simulink model "Lab_RS232_noHFC"  (Simulink 7.8)
settings: Solver=VariableStepDiscrete  StartTime=0.0  StopTime=Inf  FixedStep=Ts/4  RelTol=1e-3
PreLoadFcn:
  | clear all;
  | close all;
  | clc;
  | 
  | Txs = 1;          % Gen clk (period)
  | Trs = 1;           % Sink clk (period)
  | 
  | N = 8;    % No of characters to exchange
StartFcn:
  | clc;
  | close all;
  | 
  | TxBuffer = randi([0 255],1,N);   % Tx characters tmp array
  | RxBuffer = ones(1,N);   % Rx characters tmp array
  | 
  | RS232_Start;
StopFcn:
  | RS232_End;
  | 
  | if size(TxBuffer) == size(RxBuffer)
  |   if TxBuffer == RxBuffer
  |     disp('OK');
  |   else
  |      disp('Error');
  |      plot(TxBuffer-RxBuffer, 'o');
  |   end
  | else
  |      disp('Error: Incorrect No of characters');
  | end
libraries: simulink x1
settings Model: Creator=theodore  LastModifiedBy=theodore
settings DebuggingCC: SolverPrmCheckMsg=none

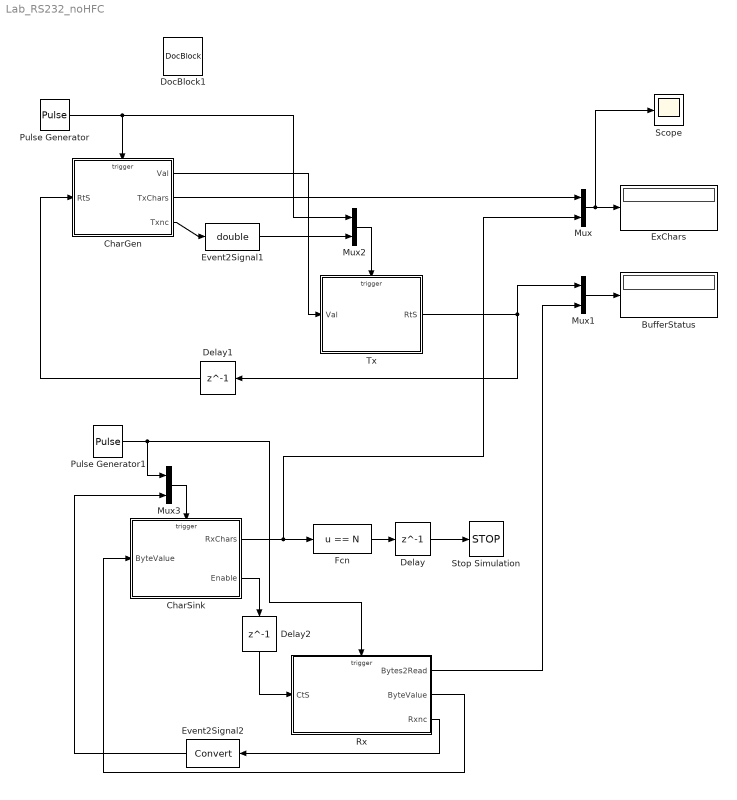
== system Lab_RS232_noHFC ==
  BufferStatus : Display
  CharGen : Stateflow chart  TreatAsAtomicUnit=on
  CharSink : Stateflow chart  TreatAsAtomicUnit=on
  Delay : Delay  DelayLength=1  SampleTime=Trs
  Delay1 : Delay  DelayLength=1  SampleTime=Trs
  Delay2 : Delay  DelayLength=1  SampleTime=Trs
  DocBlock1 : simulink/Model-Wide Utilities/DocBlock  DocumentType=Text
      content=|
      | Data exchange between two FSMs using RS232 with Tx/Rx FSMs.
      |
      | Generator stops after sending N characters.
      | Simulation stops when N characters have been received.
  Event2Signal1 : DataTypeConversion  OutDataTypeStr=double
  Event2Signal2 : DataTypeConversion
  ExChars : Display
  Fcn : Fcn  Expr=u == N
  Mux{,1..3} (4 alike) : Mux  Inputs=2
  Pulse Generator : DiscretePulseGenerator  PulseType=Time based  Period=Txs  PulseWidth=50  PhaseDelay=Txs/2
  Pulse Generator1 : DiscretePulseGenerator  PulseType=Time based  Period=Trs  PulseWidth=50  PhaseDelay=Trs/2
  Rx : Stateflow chart  TreatAsAtomicUnit=on
  Scope : Scope
  Stop Simulation : Stop
  Tx : Stateflow chart  TreatAsAtomicUnit=on
  wires:
  Pulse Generator/1 -> CharGen/Trigger, Mux2/1
  Pulse Generator1/1 -> Rx/Trigger, Mux3/1
  Fcn/1 -> Delay/1
  Mux/1 -> ExChars/1, Scope/1
  CharSink/1(RxChars) -> Mux/2, Fcn/1
  Mux1/1 -> BufferStatus/1
  CharGen/2(TxChars) -> Mux/1
  Tx/1(RtS) -> Mux1/1, Delay1/1
  CharGen/1(Val) -> Tx/1(Val)
  Mux2/1 -> Tx/Trigger
  CharGen/3(Txnc) -> Event2Signal1/1
  Event2Signal1/1 -> Mux2/2
  Delay1/1 -> CharGen/1(RtS)
  Delay/1 -> Stop Simulation/1
  Rx/1(Bytes2Read) -> Mux1/2
  Rx/2(ByteValue) -> CharSink/1(ByteValue)
  CharSink/2(Enable) -> Delay2/1
  Mux3/1 -> CharSink/Trigger
  Rx/3(Rxnc) -> Event2Signal2/1
  Event2Signal2/1 -> Mux3/2
  Delay2/1 -> Rx/1(CtS)

== stateflow chart CharGen ==
  state GenState
    en: lv++;
    Val = ml.TxBuffer[lv];
    TxChars = lv;
    Txnc;
  state IniState
    en: lv = 0;
    TxChars = lv;
  state NoAct
  (default) -> IniState
  IniState -> GenState : [RtS == 1]
  GenState -> GenState [order 1] : [RtS == 1 && lv < ml.N]
  GenState -> NoAct [order 2] : [lv == ml.N]
  data: Val output uint8 size=1; lv local double; TxChars output double; RtS input double
  events: TimeSlot input RISING_EDGE_EVENT; Txnc output EITHER_EDGE_EVENT

== stateflow chart CharSink ==
  state SinkState
    en: lv++;
    ml.RxBuffer[lv] = ByteValue;
    RxChars = lv;
    Enable = 0;
  state IniState
    en: Enable = 1;
    RxChars = lv;
  state Idle
  (default) -> IniState : {lv = 0;}
  IniState -> SinkState : Rxnc
  SinkState -> Idle [order 1] : CLK[RxChars == ml.N]
  SinkState -> IniState [order 2] : CLK
  data: lv local double; RxChars output double; ByteValue input uint8; Enable output double
  events: CLK input RISING_EDGE_EVENT; Rxnc input EITHER_EDGE_EVENT

== stateflow chart Tx ==
  state TxState
    en: ml.d2o_s1 = Val;
    ml('DOut_1');
  state IniState
  (default) -> IniState
  IniState -> TxState [order 1] : Txnc
  IniState -> IniState [order 2] : CLK{ml('B2O_1'); RtS = 1-ml.b2o_s1;}
  TxState -> IniState [order 2] : CLK{ml('B2O_1'); RtS = 1-ml.b2o_s1;}
  TxState -> TxState [order 1] : Txnc
  data: Val input uint8 size=1; RtS output double =0
  events: CLK input RISING_EDGE_EVENT; Txnc input EITHER_EDGE_EVENT

== stateflow chart Rx ==
  state SuS [parallel]
    settings: executionOrder=1
    state IniState
      Bytes2Read=0;
      IniState -> IniState : { ml('B2R_2'); Bytes2Read = ml.b2r_s2;}
    (default) -> IniState
  state DataS [parallel]
    settings: executionOrder=2
    state SinkState
      en: ml('DIn_2');
      ByteValue = ml.d2r_s2;
      lv++;
      Rxnc;
    state Idle
      lv = 0;
      Bytes2Read=0;
    Idle -> SinkState : [CtS > 0 && Bytes2Read > 0]
    (default) -> Idle
    SinkState -> Idle [order 2] : [CtS == 0]
    SinkState -> SinkState [order 1] : [CtS > 0 && Bytes2Read > 0]
  data: lv local double; Bytes2Read output double; ByteValue output uint8; CtS input double
  events: CLK input RISING_EDGE_EVENT; Rxnc output EITHER_EDGE_EVENT
